simulink model "ACS_1"  (Simulink 9.2)
settings: Solver=ode45  StartTime=0.0  StopTime=0.1  RelTol=1e-3  EnableMultiTasking=on
settings Model: Creator=Vano  LastModifiedBy=murad
settings OptimizationCC: ExpressionDepthLimit=2147483647
settings DebuggingCC: SolverPrmCheckMsg=warning

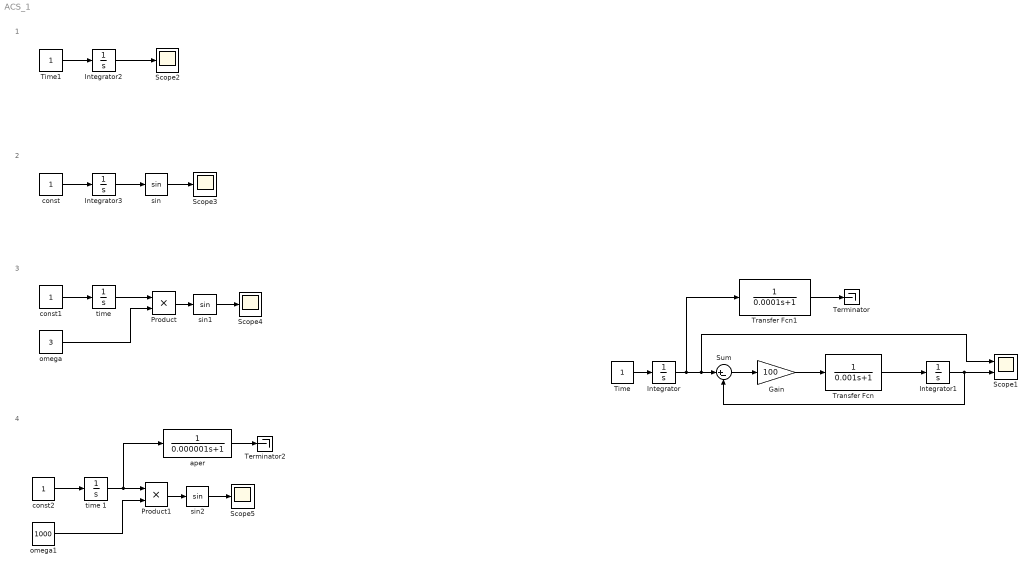
== system ACS_1 ==
  note: 1
  note: 2
  note: 3
  note: 4
  Gain : Gain  Gain=100
  Integrator{,1..3} (4 alike) : Integrator
  Product : Product
  Product1 : Product
  Scope1 : Scope  NumInputPorts=2
  Scope{2..5} (4 alike) : Scope
  Sum : Sum  Inputs=|+-
  Terminator : Terminator
  "Terminator2 " : Terminator
  Time : Constant
  Time1 : Constant
  Transfer Fcn : TransferFcn  Denominator=[0.001 1]
  Transfer Fcn1 : TransferFcn  Denominator=[0.0001 1]
  aper : TransferFcn  Denominator=[0.000001 1]
  const : Constant
  const1 : Constant
  const2 : Constant
  omega : Constant  Value=3
  omega1 : Constant  Value=1000
  "sin " : Trigonometry  OutputSignalType=real
  sin1 : Trigonometry  OutputSignalType=real
  sin2 : Trigonometry  OutputSignalType=real
  "time " : Integrator
  time 1 : Integrator
  wires:
  Transfer Fcn/1 -> Integrator1/1
  Time/1 -> Integrator/1
  Integrator/1 -> Scope1/1, Sum/1, Transfer Fcn1/1
  Sum/1 -> Gain/1
  Gain/1 -> Transfer Fcn/1
  Integrator1/1 -> Scope1/2, Sum/2
  Transfer Fcn1/1 -> Terminator/1
  Time1/1 -> Integrator2/1
  Integrator2/1 -> Scope2/1
  const/1 -> Integrator3/1
  "sin "/1 -> Scope3/1
  Integrator3/1 -> "sin "/1
  sin1/1 -> Scope4/1
  const1/1 -> "time "/1
  "time "/1 -> Product/1
  Product/1 -> sin1/1
  omega/1 -> Product/2
  omega1/1 -> Product1/2
  const2/1 -> time 1/1
  time 1/1 -> aper/1, Product1/1
  sin2/1 -> Scope5/1
  Product1/1 -> sin2/1
  aper/1 -> "Terminator2 "/1
